simulink model "AMCLIB_FW_BAM_FLT"  (Simulink 8.3)
settings: Solver=ode45  StartTime=0.0  StopTime=10.0  RelTol=1e-3
undefined symbols (not defined in the file): fltIntegGainFW, fltLambdaFW, fltPropGainFW, fltUmaxDivImax
settings Model: Creator=B37097  LastModifiedBy=B37097
settings DataIOCC: SignalLoggingSaveFormat=Dataset
settings DebuggingCC: UnderspecifiedInitializationDetection=Simplified  StateNameClashWarn=none
settings GRTTargetCC: CombineOutputUpdateFcns=on  GRTInterface=off

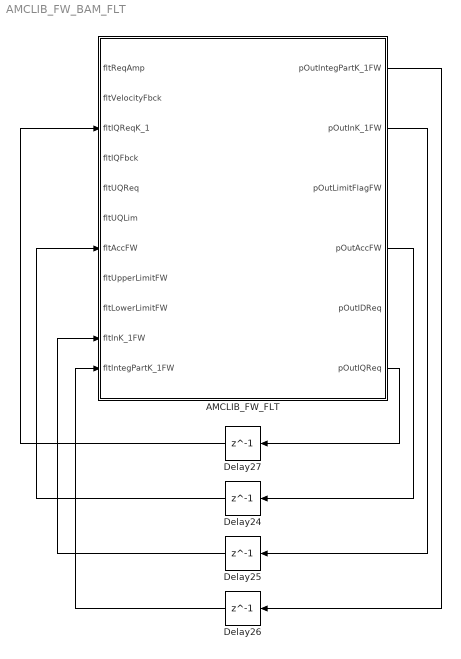
== system AMCLIB_FW_BAM_FLT ==
  AMCLIB_FW_FLT : Subsystem  mask(AMCLIB_FW_FLT){fltLambdaFW=fltLambdaFW, fltPropGainFW=fltPropGainFW, fltIntegGainFW=fltIntegGainFW, fltUmaxDivImax=fltUmaxDivImax}
      mask help: Bit accurate model of the speed loop algorithm with field weakening capability. All parameters as well as input and output values are in single precision floating data format.
      mask init:
      | pos = get_param(gcb, 'Position');width = pos(3) - pos(1); height = pos(4) - pos(2);tX=width/2;tY=height*0.9;
      mask Display: color('black');port_label('input',1,'fltReqAmp');port_label('input',2,'fltVelocityFbck');port_label('input',3,'fltIQReqK_1');port_label('input',4,'fltIQFbck');port_label('input',5,'fltUQReq');port_label('input',6,'fltUQLim');port_label('input',7,'fltAccFW');port_label('input',8,'fltUpperLimitFW');port_label('input',9,'fltLowerLimitFW');port_label('input',10,'fltInK_1FW');port_label('input',11,'fltIntegPartK_1FW');port_label('output',1,'pOutIntegPartK_1FW');port_label('output',2,'pOutInK_1FW');port_label('output',3,'pOutLimitFlagFW');port_label('output',4,'pOutAccFW');port_label('output',5,'pOutIDReq');port_label('output',6,'pOutIQReq');color('black');disp('AMCLIB_FW_FLT');color('blue');text(tX,tY, 'BAM', 'horizontalAlignment', 'center');
  Delay{24..27} (4 alike) : Delay  DelayLength=1  InitialCondition=0
  wires:
  AMCLIB_FW_FLT/6(pOutIQReq) -> Delay27/1
  Delay27/1 -> AMCLIB_FW_FLT/3(fltIQReqK_1)
  AMCLIB_FW_FLT/4(pOutAccFW) -> Delay24/1
  Delay24/1 -> AMCLIB_FW_FLT/7(fltAccFW)
  AMCLIB_FW_FLT/2(pOutInK_1FW) -> Delay25/1
  Delay25/1 -> AMCLIB_FW_FLT/10(fltInK_1FW)
  AMCLIB_FW_FLT/1(pOutIntegPartK_1FW) -> Delay26/1
  Delay26/1 -> AMCLIB_FW_FLT/11(fltIntegPartK_1FW)

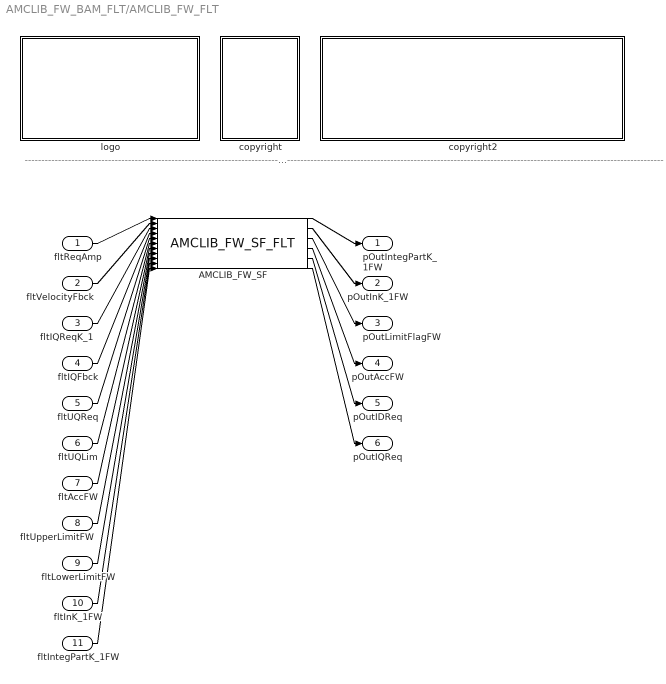
== system AMCLIB_FW_BAM_FLT/AMCLIB_FW_FLT ==
  note: ---------------------------------------------------------------------------------------------------------------------------------------------------------------------------------------------------
  fltReqAmp : Inport
  fltVelocityFbck : Inport  Port=2
  fltIQReqK_1 : Inport  Port=3
  fltIQFbck : Inport  Port=4
  fltUQReq : Inport  Port=5
  fltUQLim : Inport  Port=6
  fltAccFW : Inport  Port=7
  fltUpperLimitFW : Inport  Port=8
  fltLowerLimitFW : Inport  Port=9
  fltInK_1FW : Inport  Port=10
  fltIntegPartK_1FW : Inport  Port=11
  AMCLIB_FW_SF : S-Function  FunctionName=AMCLIB_FW_SF_FLT  Parameters=fltLambdaFW,fltPropGainFW,fltIntegGainFW,fltUmaxDivImax  EnableBusSupport=off
  copyright : Subsystem
      mask Display: text(10,90,'FILE:');text(10,75,'DESRIPTION:');text(10,60,'COPYRIGHT:');text(10,45,'VERSION:');text(10,30,'DATE:')
  copyright2 : Subsystem
      mask Display: text(10,90,'AMCLIB_FW_BAM_FLT.mdl');text(10,75,'Speed Loop with Field Weakening.');text(10,60,'NXP');text(10,45,'1.0');text(10,30,'14-Sep-2017');
  logo : Subsystem
      mask Display: image(imread('logo.jpg'))
  pOutIntegPartK_1FW : Outport
  pOutInK_1FW : Outport  Port=2
  pOutLimitFlagFW : Outport  Port=3
  pOutAccFW : Outport  Port=4
  pOutIDReq : Outport  Port=5
  pOutIQReq : Outport  Port=6
  wires:
  fltReqAmp/1 -> AMCLIB_FW_SF/1
  fltVelocityFbck/1 -> AMCLIB_FW_SF/2
  fltIQReqK_1/1 -> AMCLIB_FW_SF/3
  fltIQFbck/1 -> AMCLIB_FW_SF/4
  fltUQReq/1 -> AMCLIB_FW_SF/5
  fltUQLim/1 -> AMCLIB_FW_SF/6
  fltAccFW/1 -> AMCLIB_FW_SF/7
  fltUpperLimitFW/1 -> AMCLIB_FW_SF/8
  fltLowerLimitFW/1 -> AMCLIB_FW_SF/9
  fltInK_1FW/1 -> AMCLIB_FW_SF/10
  fltIntegPartK_1FW/1 -> AMCLIB_FW_SF/11
  AMCLIB_FW_SF/1 -> pOutIntegPartK_1FW/1
  AMCLIB_FW_SF/2 -> pOutInK_1FW/1
  AMCLIB_FW_SF/3 -> pOutLimitFlagFW/1
  AMCLIB_FW_SF/4 -> pOutAccFW/1
  AMCLIB_FW_SF/5 -> pOutIDReq/1
  AMCLIB_FW_SF/6 -> pOutIQReq/1

== system AMCLIB_FW_BAM_FLT/AMCLIB_FW_FLT/copyright ==

== system AMCLIB_FW_BAM_FLT/AMCLIB_FW_FLT/copyright2 ==

== system AMCLIB_FW_BAM_FLT/AMCLIB_FW_FLT/logo ==
